simulink model "model_T_PSH_IEEE39"  (R2020b)
settings: Solver=ode3  StartTime=0.0  StopTime=300  FixedStep=Ts  RelTol=1e-3
PostLoadFcn:
  | IEEE39BusLineLength;
  | vNomHV = 345E3;fNom=60;load('Dynamicload.mat');
InitFcn:
  | IEEE39BusLineLength;
  | vNomHV = 345E3;fNom=60;load('Dynamicload.mat');
values from neighbouring files (symbols this model uses):
  At = 1.48    [MAIN_T_PSH_IEEE39.m]
  Dturb = 0.3    [MAIN_T_PSH_IEEE39.m]
  fix_mode = 1    [MAIN_T_PSH_IEEE39.m]
  Gmax = 1    [MAIN_T_PSH_IEEE39.m]
  Gmin = 0    [MAIN_T_PSH_IEEE39.m]
  Hdam = 1    [MAIN_T_PSH_IEEE39.m]
  Kd = 1    [MAIN_T_PSH_IEEE39.m]    (also in plots_T_PSH_IEEE39.m)
  max_delay_gen2pump = 20    [MAIN_T_PSH_IEEE39.m]
  max_delay_pump2hsc = 30    [MAIN_T_PSH_IEEE39.m]
  pgen_pump = Kd*Pref    (= 0.9)    [MAIN_T_PSH_IEEE39.m]
  pgen_turb = (1-Kd)*Pref    (= 0)    [MAIN_T_PSH_IEEE39.m]
  pgen_turb_gen2pump = (1-kd_gen2pump)*Pref    (= 0)    [MAIN_T_PSH_IEEE39.m]
  pgen_turb_hsc2gen = (1-kd_hsc2gen)*Pref    (= 0.36)    [MAIN_T_PSH_IEEE39.m]
  pgen_turb_pump2hsc = (1-kd_pump2hsc)*Pref    (= 0.36)    [MAIN_T_PSH_IEEE39.m]
  Pref = 0.9    [MAIN_T_PSH_IEEE39.m]    (also in MAIN_VS_PSH.m = 1)
  qNL = 0.1    [MAIN_T_PSH_IEEE39.m]
  R = 0.04    [MAIN_T_PSH_IEEE39.m]
  r = 0.31    [MAIN_T_PSH_IEEE39.m]
  Rp = 0.05    [IEEE39BusLineLength.m]
  Sn = 320E6    (= 320000000)    [MAIN_T_PSH_IEEE39.m]
  t_gen2pump = 10    [MAIN_T_PSH_IEEE39.m]
  t_hsc2gen = 150    [MAIN_T_PSH_IEEE39.m]
  t_pump2hsc = 35    [MAIN_T_PSH_IEEE39.m]
  t_sw_off = 220    [MAIN_FS_PSH_IEEE39.m]    (also in MAIN_T_PSH_IEEE39.m; MAIN_VS_PSH.m = 45)
  t_sw_on = 130    [MAIN_FS_PSH_IEEE39.m]    (also in MAIN_T_PSH_IEEE39.m; MAIN_VS_PSH.m = 35)
  Tf = 0.05    [MAIN_T_PSH_IEEE39.m]
  Tg = 0.5    [MAIN_T_PSH_IEEE39.m]
  TL_10_11_len = 14    [IEEE39BusLineLength.m]
  TL_10_13_len = 14    [IEEE39BusLineLength.m]
  TL_13_14_len = 32    [IEEE39BusLineLength.m]
  TL_14_15_len = 70    [IEEE39BusLineLength.m]
  TL_15_16_len = 31.5    [IEEE39BusLineLength.m]
  TL_16_17_len = 26    [IEEE39BusLineLength.m]
  TL_16_19_len = 61    [IEEE39BusLineLength.m]
  TL_16_21_len = 46    [IEEE39BusLineLength.m]
  TL_16_24_len = 15    [IEEE39BusLineLength.m]
  TL_17_18_len = 26    [IEEE39BusLineLength.m]
  TL_17_27_len = 59    [IEEE39BusLineLength.m]
  TL_1_2_len = 134    [IEEE39BusLineLength.m]
  TL_1_39_len = 105    [IEEE39BusLineLength.m]
  TL_21_22_len = 47    [IEEE39BusLineLength.m]
  TL_22_23_len = 33    [IEEE39BusLineLength.m]
  TL_24_23_len = 88    [IEEE39BusLineLength.m]
  TL_25_26_len = 101    [IEEE39BusLineLength.m]
  TL_26_27_len = 46.5    [IEEE39BusLineLength.m]
  TL_26_28_len = 151    [IEEE39BusLineLength.m]
  TL_26_29_len = 200    [IEEE39BusLineLength.m]
  TL_28_29_len = 48    [IEEE39BusLineLength.m]
  TL_2_25_len = 28    [IEEE39BusLineLength.m]
  TL_2_2_len = 49    [IEEE39BusLineLength.m]
  TL_3_18_len = 42    [IEEE39BusLineLength.m]
  TL_3_4_len = 53    [IEEE39BusLineLength.m]
  TL_4_14_len = 33    [IEEE39BusLineLength.m]
  TL_4_5_len = 32.5    [IEEE39BusLineLength.m]
  TL_5_6_len = 14    [IEEE39BusLineLength.m]
  TL_5_8_len = 32    [IEEE39BusLineLength.m]
  TL_6_11_len = 26.5    [IEEE39BusLineLength.m]
  TL_6_7_len = 25.5    [IEEE39BusLineLength.m]
  TL_7_8_len = 15    [IEEE39BusLineLength.m]
  TL_8_9_len = 93    [IEEE39BusLineLength.m]
  TL_9_39_len = 136    [IEEE39BusLineLength.m]
  Tr = 6.88    [MAIN_T_PSH_IEEE39.m]
  Ts = 25e-6    (= 2.5e-05)    [MAIN_FS_PSH_IEEE39.m]    (also in MAIN_T_PSH_IEEE39.m; MAIN_VS_PSH.m = 1e-07)
  Velm = 0.05    [MAIN_T_PSH_IEEE39.m]
  Vn = 18000    [MAIN_T_PSH_IEEE39.m]
undefined symbols (not defined in the file or in its folder): D1, Delta, load15, load16, load18, load20, load21, load23, load24, load25, load26, load27, load28, load29, load3, load39, load4, load7, load8
libraries: powerlib x216, sps_avr x10, simulink_extras x7, powerlib_meascontrol x5, simulink x1
(part 4 of 9)

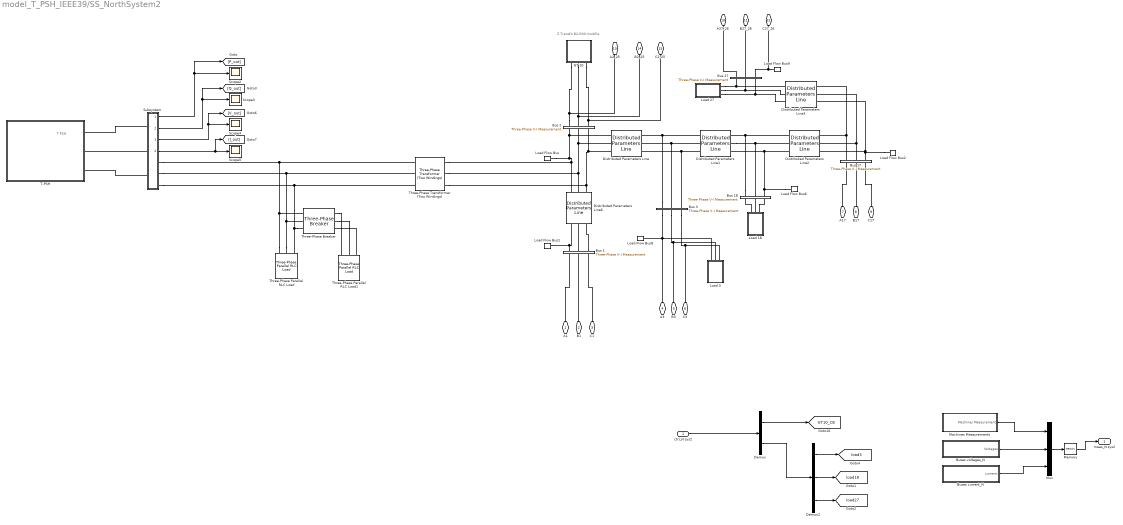
== system model_T_PSH_IEEE39/SS_NorthSystem2 ==
  note: Z Transfo B2-B30 modifie
  note: T PSH
  ctrl_N sys2 : Inport
  Bus 1 : powerlib/Measurements/Three-Phase V-I Measurement  VoltageMeasurement=phase-to-ground  SetLabelV=on  LabelV=V_bus_1  Vpu=off  VpuLL=off  CurrentMeasurement=yes  SetLabelI=on  LabelI=I_bus_1  Ipu=off  Pbase=100e6  Vbase=230e3  OutputType=Complex  PhasorSimulation=off  PSBequivalent=0
  Bus 17 : powerlib/Measurements/Three-Phase V-I Measurement  VoltageMeasurement=phase-to-ground  SetLabelV=on  LabelV=V_bus_17  Vpu=off  VpuLL=off  CurrentMeasurement=yes  SetLabelI=on  LabelI=I_bus_17  Ipu=off  Pbase=100e6  Vbase=230e3  OutputType=Complex  PhasorSimulation=off  PSBequivalent=0
  Bus 18 : powerlib/Measurements/Three-Phase V-I Measurement  VoltageMeasurement=phase-to-ground  SetLabelV=on  LabelV=V_bus_18  Vpu=off  VpuLL=off  CurrentMeasurement=yes  SetLabelI=on  LabelI=I_bus_18  Ipu=off  Pbase=100e6  Vbase=230e3  OutputType=Complex  PhasorSimulation=off  PSBequivalent=0
  Bus 2 : powerlib/Measurements/Three-Phase V-I Measurement  VoltageMeasurement=phase-to-ground  SetLabelV=on  LabelV=V_bus_2  Vpu=off  VpuLL=off  CurrentMeasurement=yes  SetLabelI=on  LabelI=I_bus_2  Ipu=off  Pbase=100e6  Vbase=230e3  OutputType=Complex  PhasorSimulation=off  PSBequivalent=0
  Bus 27 : powerlib/Measurements/Three-Phase V-I Measurement  VoltageMeasurement=phase-to-ground  SetLabelV=on  LabelV=V_bus_27  Vpu=off  VpuLL=off  CurrentMeasurement=yes  SetLabelI=on  LabelI=I_bus_27  Ipu=off  Pbase=100e6  Vbase=230e3  OutputType=Complex  PhasorSimulation=off  PSBequivalent=0
  Bus 3 : powerlib/Measurements/Three-Phase V-I Measurement  VoltageMeasurement=phase-to-ground  SetLabelV=on  LabelV=V_bus_3  Vpu=off  VpuLL=off  CurrentMeasurement=yes  SetLabelI=on  LabelI=I_bus_3  Ipu=off  Pbase=100e6  Vbase=230e3  OutputType=Complex  PhasorSimulation=off  PSBequivalent=0
  Buses current_N : Subsystem
  Buses voltages_N : Subsystem
  Demux : Demux  Outputs=[1 6]
  Demux2 : Demux  Outputs=[2 2 2]
  Distributed Parameters Line : powerlib/Elements/Distributed Parameters Line  Phases=3  Length=TL_2_2_len  Frequency=fNom  Resistance=[1.547 6.189]/TL_2_2_len  Inductance="[0.048  0.143]/TL_2_2_len"  Capacitance=[0.573e-6 0.261e-6]/TL_2_2_len  x1=[-0.0002 -9.01675283131685e-09 0 0;-0.000175 -9.03116162920668e-09 162254.642108417 -193092.745434423;-0.00015 -9.04476822710152e-09 164067.253485419 -191554.977392481;-0.000125 -9.05757141638467e-09 165865.291460313 -190000.194329857;-0.0001 -9.06957005980283e-09 167648.596320969 -188428.534351372;-7.5e-05 -9.08076309156712e-09 169417.00966394 -186840.137060953;-5e-05 -9.09114951744772e-09 171170.374408526 -185235.143549232;-2.5e-05 -9.10072841486225e-09 172908.534810733 -183613.696381013]  x2=[-0.0002 2.00645197588943e-09 0 0;-0.000175 1.87438018048954e-09 136418.087730126 -205057.992053123;-0.00015 1.74214189180416e-09 138344.61519234 -203763.19275921;-0.000125 1.60974885600272e-09 140258.85408591 -202450.294040337;-0.0001 1.47721283300015e-09 142160.634377069 -201119.412515759;-7.5e-05 1.34454559541237e-09 144049.787138696 -199770.666402069;-5e-05 1.21175892751051e-09 145926.14456532 -198404.175502695;-2.5e-05 1.07886462417419e-09 147789.539988023 -197020.06119726]  x3=[-0.0002 2.38791880701982e-10 0 0;-0.000175 2.4040678801237e-10 -238.391238439602 676.648615683037;-0.00015 2.42000341001791e-10 -244.757858873933 674.371841084138;-0.000125 2.43572398121653e-10 -251.102738500023 672.035164879028;-0.0001 2.45122819732755e-10 -257.425313728979 669.638794624799;-7.5e-05 2.46651468117683e-10 -263.72502295311 667.182943180912;-5e-05 2.48158207493049e-10 -270.001306595819 664.667828690293;-2.5e-05 2.4964290402155e-10 -276.2536071613 662.093674559954]  x4=[-0.0002 -2.46531065369881e-10 0 0;-0.000175 -2.48327425885902e-10 1223.29475249095 -2078.96610672438;-0.00015 -2.50101728524102e-10 1242.83388654417 -2067.34468784689;-0.000125 -2.51853815680662e-10 1262.26262490541 -2055.53963546064;-0.0001 -2.53583531725068e-10 1281.57924180177 -2043.55199815863;-7.5e-05 -2.55290723013941e-10 1300.78202141965 -2031.38284075212;-5e-05 -2.56975237904679e-10 1319.86925805714 -2019.03324417604;-2.5e-05 -2.5863692676893e-10 1338.83925627551 -2006.50430539295]  x5=0.000193191614724863  V1=ones(3,3)  V2=ones(3,3)  I1=ones(3,3)  I2=ones(3,3)  nHarmo=1  Measurements=None  Decoupling=off  VsMag0=0  VrMag0=0  VsAngle0=0  VrAngle0=0  IsMag0=0  IrMag0=0  IsAngle0=0  IrAngle0=0
  Distributed Parameters Line1 : powerlib/Elements/Distributed Parameters Line  Phases=3  Length=TL_3_18_len  Frequency=fNom  Resistance=[1.309 5.237]/TL_3_18_len  Inductance=[0.042 0.126]/TL_3_18_len  Capacitance=[0.476e-6 0.217e-6]/TL_3_18_len  x1=[-0.000175 1.87438018048954e-09 136418.087730126 -205057.992053123;-0.00015 1.74214189180416e-09 138344.61519234 -203763.19275921;-0.000125 1.60974885600272e-09 140258.85408591 -202450.294040337;-0.0001 1.47721283300015e-09 142160.634377069 -201119.412515759;-7.5e-05 1.34454559541237e-09 144049.787138696 -199770.666402069;-5e-05 1.21175892751051e-09 145926.14456532 -198404.175502695;-2.5e-05 1.07886462417419e-09 147789.539988023 -197020.06119726]  x2=[-0.000175 1.5591113079116e-08 127087.178338194 -211171.403878634;-0.00015 1.54196628970743e-08 129071.737261978 -209964.273522979;-0.000125 1.5246843051416e-08 131044.831287754 -208738.492926515;-0.0001 1.50726688929991e-08 133006.2851539 -207494.170970163;-7.5e-05 1.48971558929795e-08 134955.924632742 -206231.418181793;-5e-05 1.47203196414366e-08 136893.576546031 -204950.346726409;-2.5e-05 1.45421758459888e-08 138819.068780318 -203651.070396186]  x3=[-0.000175 1.19211576192778e-10 8.2739916519236 -147.595530559831;-0.00015 1.21633098360464e-10 9.66462301857463 -147.510971877278;-0.000125 1.24043816373058e-10 11.0543959175273 -147.41331041728;-0.0001 1.26443516096648e-10 12.443186901117 -147.302554854692;-7.5e-05 1.28831984376029e-10 13.8308726088984 -147.178715027463;-5e-05 1.31209009053639e-10 15.2173297786031 -147.041801935764;-2.5e-05 1.33574378988401e-10 16.6024352570888 -146.891827741006]  x4=[-0.000175 -9.47057273450053e-11 838.617573044516 -1272.61392020957;-0.00015 -9.75021136474352e-11 850.574214877113 -1264.65375230151;-0.000125 -1.00289839248364e-10 862.455303789839 -1256.58125053482;-0.0001 -1.03068656525885e-10 874.25978443568 -1248.39713195578;-7.5e-05 -1.05838318649379e-10 885.986608272409 -1240.10212352512;-5e-05 -1.08598579601444e-10 897.634733655728 -1231.69696205346;-2.5e-05 -1.1134919419974e-10 909.203125931789 -1223.18239413583]  x5=0.000165354165354248  V1=ones(3,3)  V2=ones(3,3)  I1=ones(3,3)  I2=ones(3,3)  nHarmo=1  Measurements=None  Decoupling=off  VsMag0=0  VrMag0=0  VsAngle0=0  VrAngle0=0  IsMag0=0  IrMag0=0  IsAngle0=0  IrAngle0=0
  Distributed Parameters Line2 : powerlib/Elements/Distributed Parameters Line  Phases=3  Length=TL_17_18_len  Frequency=fNom  Resistance=[0.833 3.333]/TL_17_18_len  Inductance=[0.026 0.078]/TL_17_18_len  Capacitance=[0.294e-6 0.134e-6]/TL_17_18_len  x1=[-0.000125 1.5246843051416e-08 0 0;-0.0001 1.50726688929991e-08 133006.2851539 -207494.170970163;-7.5e-05 1.48971558929795e-08 134955.924632742 -206231.418181793;-5e-05 1.47203196414366e-08 136893.576546031 -204950.346726409;-2.5e-05 1.45421758459888e-08 138819.068780318 -203651.070396186]  x2=[-0.000125 2.39408399520577e-08 0 0;-0.0001 2.36824783705596e-08 131020.122877065 -208712.127601341;-7.5e-05 2.34220131743981e-08 132981.329601984 -207468.039590694;-5e-05 2.31594674995981e-08 134930.724156296 -206205.523069169;-2.5e-05 2.28948646669843e-08 136868.133383506 -204924.690180784]  x3=[-0.000125 3.50356367901172e-10 0 0;-0.0001 3.52540545204145e-10 294.543982123679 -513.169742251818;-7.5e-05 3.54693407817469e-10 299.367306278856 -510.370953263216;-5e-05 3.56814764511438e-10 304.164038898918 -507.52683017553;-2.5e-05 3.58904426854883e-10 308.933753910338 -504.637625620217]  x4=[-0.000125 -2.97929795960239e-10 0 0;-0.0001 -3.00664277176283e-10 568.397230248573 -898.079002636142;-7.5e-05 -3.03372051652758e-10 576.836017265337 -892.682198069237;-5e-05 -3.06052878869477e-10 585.223566371725 -887.206100307922;-2.5e-05 -3.08706520699866e-10 593.559132537125 -881.651195770863]  x5=0.000102235023353056  V1=ones(3,3)  V2=ones(3,3)  I1=ones(3,3)  I2=ones(3,3)  nHarmo=1  Measurements=None  Decoupling=off  VsMag0=0  VrMag0=0  VsAngle0=0  VrAngle0=0  IsMag0=0  IrMag0=0  IsAngle0=0  IrAngle0=0
  Distributed Parameters Line3 : powerlib/Elements/Distributed Parameters Line  Phases=3  Length=TL_17_27_len  Frequency=fNom  Resistance=[1.547 6.189]/TL_17_27_len  Inductance=[0.055 0.164]/TL_17_27_len  Capacitance=[0.717e-6 0.326e-6]/TL_17_27_len  x1=[-0.00025 1.57832792261442e-08 0 0;-0.000225 1.55059702220527e-08 0 0;-0.0002 1.52272838880291e-08 125254.843954793 -212986.10664044;-0.000175 1.49472449786049e-08 127256.586831929 -211796.164829682;-0.00015 1.46658783684552e-08 129247.026043211 -210587.410058936;-0.000125 1.43832090501892e-08 131225.984786321 -209359.949696791;-0.0001 1.40992621321302e-08 133193.287278701 -208113.892773374;-7.5e-05 1.38140628360853e-08 135148.758773167 -206849.349970666;-5e-05 1.3527636495105e-08 137092.225573436 -205566.433612669;-2.5e-05 1.3240008551233e-08 139023.515049548 -204265.257655433]  x2=[-0.00025 2.52002970722805e-08 0 0;-0.000225 2.49527939935447e-08 0 0;-0.0002 2.47030744633669e-08 123060.673798531 -213502.009152357;-0.000175 2.44511606632795e-08 125067.376889071 -212332.723740496;-0.00015 2.4197074969723e-08 127062.970772043 -211144.577708384;-0.000125 2.39408399520577e-08 129047.278187261 -209937.67659402;-0.0001 2.36824783705596e-08 131020.122877065 -208712.127601341;-7.5e-05 2.34220131743981e-08 132981.329601984 -207468.039590694;-5e-05 2.31594674995981e-08 134930.724156296 -206205.523069169;-2.5e-05 2.28948646669843e-08 136868.133383506 -204924.690180784]  x3=[-0.00025 -1.30695208352182e-11 0 0;-0.000225 -1.19699239755897e-11 0 0;-0.0002 -1.08692638781025e-11 389.105924626069 -679.477744299816;-0.000175 -9.76763830975041e-12 395.492439326144 -675.780355407322;-0.00015 -8.6651451232862e-12 401.843824100982 -672.02293979623;-0.000125 -7.5618822485294e-12 408.159514783861 -668.205831221921;-0.0001 -6.45794768366773e-12 414.438950378618 -664.32936874205;-7.5e-05 -5.35343948655229e-12 420.681573109475 -660.393896686428;-5e-05 -4.24845576598752e-12 426.886828470585 -656.399764626439;-2.5e-05 -3.14309467301663e-12 433.054165275288 -652.347327343986]  x4=[-0.00025 7.33109579138771e-11 0 0;-0.000225 7.15189673862492e-11 0 0;-0.0002 6.97206241304082e-11 446.204587923734 -887.439579923524;-0.000175 6.79160878856002e-11 454.548524901683 -883.194874840398;-0.00015 6.61055189411687e-11 462.852086251406 -878.871719281768;-0.000125 6.42890781223161e-11 471.11453440257 -874.470497255306;-0.0001 6.24669267758187e-11 479.335135436757 -869.991599703001;-7.5e-05 6.0639226755695e-11 487.513159152651 -865.435424466433;-5e-05 5.88061404088289e-11 495.647879130899 -860.802376251428;-2.5e-05 5.69678305605486e-11 503.738572798637 -856.09286659212]  x5=0.000231222836242444  V1=ones(3,3)  V2=ones(3,3)  I1=ones(3,3)  I2=ones(3,3)  nHarmo=1  Measurements=None  Decoupling=off  VsMag0=0  VrMag0=0  VsAngle0=0  VrAngle0=0  IsMag0=0  IrMag0=0  IsAngle0=0  IrAngle0=0
  Distributed Parameters Line6 : powerlib/Elements/Distributed Parameters Line  Phases=3  Length=TL_1_2_len  Frequency=fNom  Resistance=[4.166 16.66]/TL_1_2_len  Inductance=[0.13 0.389]/TL_1_2_len  Capacitance=[1.56e-6 0.708e-6]/TL_1_2_len  x1=[-0.000525 -8.75711731874504e-09 251976.802401335 -10914.1188870031;-0.0005 -8.78181248505178e-09 251862.744448447 -13288.4139122704;-0.000475 -8.80572759999627e-09 251726.314590302 -15661.528583779;-0.00045 -8.82886053929973e-09 251567.524945388 -18033.2521077623;-0.000425 -8.85120924816073e-09 251386.38961832 -20403.3738140233;-0.0004 -8.87277174143772e-09 251182.924698584 -22771.6831746477;-0.000375 -8.89354610382539e-09 250957.148259112 -25137.9698227045;-0.00035 -8.91353049002474e-09 250709.080354672 -27502.0235709313;-0.000325 -8.93272312490704e-09 250438.74302009 -29863.6344304052;-0.0003 -8.95112230367148e-09 250146.160268291 -32222.5926291943;-0.000275 -8.96872639199662e-09 249831.358088167 -34578.6886309919;-0.00025 -8.98553382618555e-09 249494.364442267 -36931.7131537278;-0.000225 -9.00154311330477e-09 249135.209264316 -39281.4571881585;-0.0002 -9.01675283131685e-09 248753.924456554 -41627.7120164325;-0.000175 -9.03116162920668e-09 248350.543886901 -43970.2692306296;-0.00015 -9.04476822710152e-09 247925.103385952 -46308.920751273;-0.000125 -9.05757141638467e-09 247477.640743792 -48643.4588458125;-0.0001 -9.06957005980283e-09 247008.195706642 -50973.676147076;-7.5e-05 -9.08076309156712e-09 246516.809973322 -53299.3656716892;-5e-05 -9.09114951744772e-09 246003.527191556 -55620.3208384611;-2.5e-05 -9.10072841486225e-09 245468.392954087 -57936.3354867339]  x2=[-0.000525 -6.75393890925529e-12 252971.338182445 4089.24039293867;-0.0005 -3.92179325042561e-11 252998.636955303 1704.9063062137;-0.000475 -7.167844253573e-11 253003.462926364 -679.579220147331;-0.00045 -1.04132585673486e-10 252985.815666956 -3064.00438235263;-0.000425 -1.36577479152877e-10 252945.696744611 -5448.1573819723;-0.0004 -1.69010241030865e-10 252883.109722924 -7831.82644475151;-0.000375 -2.01427990442011e-10 252798.060161236 -10214.7998394215;-0.00035 -2.33827847854369e-10 252690.555614141 -12596.8658965068;-0.000325 -2.66206935325264e-10 252560.605630813 -14977.8130271267;-0.0003 -2.98562376756929e-10 252408.221754163 -17357.4297417904;-0.000275 -3.30891298151972e-10 252233.417519807 -19735.504669182;-0.00025 -3.63190827868667e-10 252036.208454868 -22111.8265749363;-0.000225 -3.95458096876025e-10 251816.612076595 -24486.1843804013;-0.0002 -4.27690239008639e-10 251574.647890809 -26858.3671813882;-0.000175 -4.59884391221277e-10 251310.337390167 -29228.1642669041;-0.00015 -4.92037693843189e-10 251023.704052257 -31595.3651378698;-0.000125 -5.24147290832123e-10 250714.773337508 -33959.7595258162;-0.0001 -5.56210330028012e-10 250383.572686934 -36321.1374115629;-7.5e-05 -5.88223963406325e-10 250030.13151969 -38679.2890438722;-5e-05 -6.20185347331038e-10 249654.481230466 -41034.0049580811;-2.5e-05 -6.52091642807227e-10 249256.655186692 -43385.075994707]  x3=[-0.000525 9.86559548328332e-13 565.12948251465 82.0573040008989;-0.0005 1.48814824191351e-12 565.877736710338 76.7275637061704;-0.000475 1.98960474956722e-12 566.57572637349 71.391008025587;-0.00045 2.49088452902299e-12 567.223389504627 66.0481109828808;-0.000425 2.99194305371233e-12 567.820668574566 60.6993471650603;-0.0004 3.49273581671994e-12 568.367510529526 55.3451916802549;-0.000375 3.99321833473695e-12 568.863866795843 49.986120115513;-0.00035 4.49334615201228e-12 569.309693284283 44.6226084945576;-0.000325 4.99307484430142e-12 569.70495039396 39.2551332355034;-0.0003 5.49236002281242e-12 570.049603015852 33.8841711085381;-0.000275 5.99115733814882e-12 570.343620535919 28.5101991935732;-0.00025 6.48942248424897e-12 570.586976837827 23.1336948378672;-0.000225 6.98711120232157e-12 570.77965030526 17.7551356136242;-0.0002 7.48417928477701e-12 570.921623823849 12.3749992755742;-0.000175 7.9805825791541e-12 571.012884782683 6.99376371853492;-0.00015 8.47627699204198e-12 571.053425075437 1.61190693496356;-0.000125 8.97121849299674e-12 571.043241101087 -3.77009302750197;-0.0001 9.46536311845247e-12 570.982333764234 -9.15175810850574;-7.5e-05 9.95866697562633e-12 570.870708475019 -14.5326102774379;-5e-05 1.04510862464174e-11 570.708375148644 -19.9121715758963;-2.5e-05 1.09425771912989e-11 570.495348204497 -25.2899641601411]  x4=[-0.000525 -1.13789397052226e-11 1167.19515497174 42.3240124393784;-0.0005 -1.19704871209246e-11 1167.54218087574 31.3217718787318;-0.000475 -1.2560971248746e-11 1167.78549893238 20.3167491372014;-0.00045 -1.31503396384722e-11 1167.92508752875 9.30992174453907;-0.000425 -1.37385399389952e-11 1167.9609342658 -1.69773260920349;-0.0004 -1.43255199029632e-11 1167.89303595939 -12.7052361605192;-0.000375 -1.49112273914218e-11 1167.72139864065 -23.7116111592963;-0.00035 -1.54956103784453e-11 1167.4460375554 -34.7158799556672;-0.000325 -1.60786169557578e-11 1167.06697716281 -45.7170650868498;-0.0003 -1.66601953373442e-11 1166.58425113321 -56.7141893639707;-0.000275 -1.72402938640497e-11 1165.99790234511 -67.7062759588652;-0.00025 -1.78188610081691e-11 1165.30798288141 -78.6923484908445;-0.000225 -1.83958453780234e-11 1164.51455402475 -89.6714311134237;-0.0002 -1.89711957225245e-11 1163.61768625205 -100.642548601002;-0.000175 -1.95448609357282e-11 1162.61745922831 -111.604726435489;-0.00015 -2.01167900613733e-11 1161.51396179947 -122.556990892864;-0.000125 -2.06869322974078e-11 1160.30729198455 -133.49836912967;-0.0001 -2.12552370005017e-11 1158.99755696695 -144.42788926943;-7.5e-05 -2.18216536905453e-11 1157.58487308489 -155.344580488969;-5e-05 -2.23861320551331e-11 1156.06936582114 -166.24747310465;-2.5e-05 -2.2948621954033e-11 1154.4511697918 -177.135598658511]  x5=0.000524797103650544  V1=ones(3,3)  V2=ones(3,3)  I1=ones(3,3)  I2=ones(3,3)  nHarmo=1  Measurements=None  Decoupling=off  VsMag0=0  VrMag0=0  VsAngle0=0  VrAngle0=0  IsMag0=0  IrMag0=0  IsAngle0=0  IrAngle0=0
  GT 10 : Subsystem
  Load 18 : Subsystem  SystemSampleTime=20e-3
  Load 27 : Subsystem  SystemSampleTime=20e-3
  Load 3 : Subsystem  SystemSampleTime=20e-3
  Load Flow Bus : powerlib/Measurements/Load Flow Bus  LConnTagsString=a  Phases=single  Connectors=on one side  ID=Bus-2  Vbase=345e+003  Vref=1  Vangle=0  VLF=1.028  VLFb=1  VLFc=1  angleLF=24.05  angleLFb=0  angleLFc=0
      settings: AttributesFormatString=%<ID>\n%<Vbase>V\n%<VLF>pu\n%<angleLF>deg.
  Load Flow Bus1 : powerlib/Measurements/Load Flow Bus  LConnTagsString=a  Phases=single  Connectors=on one side  ID=Bus-1  Vbase=345e+003  Vref=1  Vangle=0  VLF=1.036  VLFb=1  VLFc=1  angleLF=22.64  angleLFb=0  angleLFc=0
      settings: AttributesFormatString=%<ID>\n%<Vbase>V\n%<VLF>pu\n%<angleLF>deg.
  Load Flow Bus2 : powerlib/Measurements/Load Flow Bus  LConnTagsString=a  Phases=single  Connectors=on one side  ID=Bus-17  Vbase=345e+003  Vref=1  Vangle=0  VLF=1.01  VLFb=1  VLFc=1  angleLF=19.53  angleLFb=0  angleLFc=0
      settings: AttributesFormatString=%<ID>\n%<Vbase>V\n%<VLF>pu\n%<angleLF>deg.
  Load Flow Bus6 : powerlib/Measurements/Load Flow Bus  LConnTagsString=a  Phases=single  Connectors=on one side  ID=Bus-18  Vbase=345e+003  Vref=1  Vangle=0  VLF=1.009  VLFb=1  VLFc=1  angleLF=19.72  angleLFb=0  angleLFc=0
      settings: AttributesFormatString=%<ID>\n%<Vbase>V\n%<VLF>pu\n%<angleLF>deg.
  Load Flow Bus8 : powerlib/Measurements/Load Flow Bus  LConnTagsString=a  Phases=single  Connectors=on one side  ID=Bus-3  Vbase=345e+003  Vref=1  Vangle=0  VLF=1.01  VLFb=1  VLFc=1  angleLF=21  angleLFb=0  angleLFc=0
      settings: AttributesFormatString=%<ID>\n%<Vbase>V\n%<VLF>pu\n%<angleLF>deg.
  Load Flow Bus9 : powerlib/Measurements/Load Flow Bus  LConnTagsString=a  Phases=single  Connectors=on one side  ID=Bus-27  Vbase=345e+003  Vref=1  Vangle=0  VLF=1.013  VLFb=1  VLFc=1  angleLF=19.76  angleLFb=0  angleLFc=0
      settings: AttributesFormatString=%<ID>\n%<Vbase>V\n%<VLF>pu\n%<angleLF>deg.
  Machines Measurements : Subsystem
      mask Display: disp('Machines Measurements')
  Memory : Memory
  Mux : Mux  Inputs=3
  Scope{2..5} (4 alike) : Scope
  Subsystem : Subsystem
  T-PSH : Subsystem
  Three-Phase Parallel RLC Load : powerlib/Elements/Three-Phase Parallel RLC Load  LConnTagsString=A|B|C  Configuration=Y (grounded)  NominalVoltage=18e3  Vabc=[1e3 1e3 1e3]  Vabcp=[1e3 1e3 1e3]  NominalFrequency=60  UnbalancedPower=off  ActivePower=0.001e6  InductivePower=0  CapacitivePower=0  Pabc=[10e3 9e3 11e3]  QLabc=[100 90 110]  QCabc=[100 90 110]  Pabcp=[10e3 9e3 11e3]  QLabcp=[100 90 110]  QCabcp=[100 90 110]  Measurements=None  LoadType=constant Z
  Three-Phase Parallel RLC Load1 : powerlib/Elements/Three-Phase Parallel RLC Load  LConnTagsString=A|B|C  Configuration=Y (grounded)  NominalVoltage=18e3  Vabc=[1e3 1e3 1e3]  Vabcp=[1e3 1e3 1e3]  NominalFrequency=60  UnbalancedPower=off  ActivePower=300e6  InductivePower=0  CapacitivePower=0  Pabc=[10e3 9e3 11e3]  QLabc=[100 90 110]  QCabc=[100 90 110]  Pabcp=[10e3 9e3 11e3]  QLabcp=[100 90 110]  QCabcp=[100 90 110]  Measurements=None  LoadType=constant Z
  Three-Phase Transformer (Two Windings) : powerlib/Elements/Three-Phase Transformer (Two Windings)  Winding1Connection=Yg  Winding2Connection=Yg  CoreType=Three single-phase transformers  SetSaturation=off  Hysteresis=off  DataFile='hysteresis'  SetInitialFlux=off  Measurements=None  UNITS=pu  NominalPower=[1000e6 , 60 ]  Winding1=[18e3 , 0.002 , 0.08 ]  Winding2=[ 345e3 , 0.002 , 0.08 ]  Rm=500  Lm=500  L0=0.5  Saturation=[ 0,0 ; 0.0024,1.2 ; 1.0,1.52 ]  InitialFluxes=[ 0.8 , -0.8 , 0.7 ]  BreakLoop=off  DiscreteSolver=Trapezoidal iterative  DataType=off  TransfoNumber=1
  Three-Phase Breaker : powerlib/Elements/Three-Phase Breaker  InitialState=open  SwitchA=on  SwitchB=on  SwitchC=on  SwitchTimes=[t_sw_on t_sw_off]  External=off  BreakerResistance=0.01  SnubberResistance=1e6  SnubberCapacitance=inf  Measurements=None
  A1 : PMIOPort  Side=Left
  B1 : PMIOPort  Port=2  Side=Left
  C1 : PMIOPort  Port=3  Side=Left
  A3 : PMIOPort  Port=4  Side=Left
  B3 : PMIOPort  Port=5  Side=Left
  C3 : PMIOPort  Port=6  Side=Left
  A17 : PMIOPort  Port=7  Side=Left
  B17 : PMIOPort  Port=8  Side=Left
  C17 : PMIOPort  Port=9  Side=Left
  A27_26 : PMIOPort  Port=10  Side=Right
  B27_26 : PMIOPort  Port=11  Side=Right
  C27_26 : PMIOPort  Port=12  Side=Right
  A2_25 : PMIOPort  Port=13  Side=Right
  B2_25 : PMIOPort  Port=14  Side=Right
  C2_25 : PMIOPort  Port=15  Side=Right
  meas_N sys2 : Outport
  tag scope: GT10_CB=global, load18=global, load27=global, load3=global
  wires:
  Machines Measurements/1(Machines Measurements) -> Mux/1
  Mux/1 -> Memory/1
  Memory/1 -> meas_N sys2/1
  Buses voltages_N/1(Voltages) -> Mux/2
  Buses current_N/1(curremt) -> Mux/3
  Demux/2 -> Demux2/1
  Demux/1 -> [GT10_CB]
  Demux2/1 -> [load3]
  Demux2/3 -> [load27]
  Demux2/2 -> [load18]
  ctrl_N sys2/1 -> Demux/1
  Subsystem/1(Out1) -> [P_out], Scope2/1
  Subsystem/2(Out2) -> [Q_out], Scope3/1
  Subsystem/3(Out3) -> [V_out], Scope4/1
  Subsystem/4(Out4) -> [I_out], Scope5/1
  connections:
  Load 27/LConn3 -- Distributed Parameters Line3/LConn3 -- Bus 27/LConn3
  Load 27/LConn2 -- Distributed Parameters Line3/LConn2 -- Bus 27/LConn2
  Load 27/LConn1 -- Distributed Parameters Line3/LConn1 -- Bus 27/LConn1
  GT 10/RConn3 -- C2_25/RConn1 -- Bus 2/RConn3
  GT 10/RConn2 -- B2_25/RConn1 -- Bus 2/RConn2
  Bus 2/RConn1 -- GT 10/RConn1 -- A2_25/RConn1
  Load 18/LConn3 -- Bus 18/LConn3
  Load 18/LConn2 -- Bus 18/LConn2
  Load 18/LConn1 -- Bus 18/LConn1
  Load Flow Bus2/LConn1 -- Distributed Parameters Line2/RConn3 -- Distributed Parameters Line3/RConn3 -- Bus 17/RConn3
  Distributed Parameters Line2/RConn2 -- Distributed Parameters Line3/RConn2 -- Bus 17/RConn2
  Distributed Parameters Line2/RConn1 -- Distributed Parameters Line3/RConn1 -- Bus 17/RConn1
  Bus 1/RConn3 -- Distributed Parameters Line6/RConn1
  Bus 1/RConn2 -- Distributed Parameters Line6/RConn2
  Load Flow Bus1/LConn1 -- Distributed Parameters Line6/RConn3 -- Bus 1/RConn1
  Bus 2/LConn3 -- Distributed Parameters Line6/LConn1 -- Three-Phase Transformer (Two Windings)/RConn3 -- Distributed Parameters Line/LConn3
  Distributed Parameters Line6/LConn3 -- Three-Phase Transformer (Two Windings)/RConn1 -- Load Flow Bus/LConn1 -- Distributed Parameters Line/LConn1 -- Bus 2/LConn1
  Distributed Parameters Line/RConn2 -- Distributed Parameters Line1/LConn2 -- Bus 3/RConn2
  Bus 3/RConn1 -- Distributed Parameters Line1/LConn1 -- Distributed Parameters Line/RConn1
  Distributed Parameters Line/RConn3 -- Bus 3/RConn3 -- Distributed Parameters Line1/LConn3
  Bus 3/LConn3 -- C3/RConn1 -- Load 3/LConn3
  Bus 3/LConn2 -- B3/RConn1 -- Load 3/LConn2
  Load Flow Bus8/LConn1 -- Load 3/LConn1 -- Bus 3/LConn1 -- A3/RConn1
  Bus 2/LConn2 -- Distributed Parameters Line6/LConn2 -- Three-Phase Transformer (Two Windings)/RConn2 -- Distributed Parameters Line/LConn2
  B1/RConn1 -- Bus 1/LConn2
  A1/RConn1 -- Bus 1/LConn1
  C1/RConn1 -- Bus 1/LConn3
  Bus 18/RConn1 -- Distributed Parameters Line1/RConn1 -- Distributed Parameters Line2/LConn1
  Bus 18/RConn2 -- Distributed Parameters Line1/RConn2 -- Distributed Parameters Line2/LConn2
  Load Flow Bus6/LConn1 -- Distributed Parameters Line1/RConn3 -- Distributed Parameters Line2/LConn3 -- Bus 18/RConn3
  Bus 17/LConn2 -- B17/RConn1
  Bus 17/LConn3 -- C17/RConn1
  Bus 17/LConn1 -- A17/RConn1
  Bus 27/RConn2 -- B27_26/RConn1
  Load Flow Bus9/LConn1 -- Bus 27/RConn3 -- C27_26/RConn1
  Bus 27/RConn1 -- A27_26/RConn1
  Three-Phase Breaker/LConn3 -- Three-Phase Parallel RLC Load/LConn3 -- Three-Phase Transformer (Two Windings)/LConn3 -- Subsystem/RConn3
  Three-Phase Parallel RLC Load/LConn2 -- Three-Phase Transformer (Two Windings)/LConn2 -- Subsystem/RConn2 -- Three-Phase Breaker/LConn2
  Three-Phase Parallel RLC Load/LConn1 -- Three-Phase Breaker/LConn1 -- Three-Phase Transformer (Two Windings)/LConn1 -- Subsystem/RConn1
  Subsystem/LConn1 -- T-PSH/RConn1
  Three-Phase Breaker/RConn1 -- Three-Phase Parallel RLC Load1/LConn1
  Subsystem/LConn3 -- T-PSH/RConn3
  Three-Phase Parallel RLC Load1/LConn3 -- Three-Phase Breaker/RConn3
  Subsystem/LConn2 -- T-PSH/RConn2
  Three-Phase Breaker/RConn2 -- Three-Phase Parallel RLC Load1/LConn2
